simulink model "analysis_PI_ctrl_lin_model_z"  (R2020b)
settings: Solver=VariableStepAuto  StartTime=0.0  StopTime=10.0  RelTol=1e-3
values from neighbouring files (symbols this model uses):
  B = 10    [hinfCostFunc.m]    (also in hinf_analysis_z.m; hinf_cmd_lmi.m = [zeros(4,2); Sigma.B]; init_rob_synth_sim.m; muCostFunc.m = 11)
  dq0 = [0;0;0]    [hinfCostFunc.m]    (also in hinf_analysis_z.m; init_rob_synth_sim.m = [0; 0; 0]; muCostFunc.m; mu_analysis_z.m)
  ev0 = [0;0;0]    [hinfCostFunc.m]    (also in hinf_analysis_z.m; muCostFunc.m; mu_analysis_z.m)
  K = 150    [hinfCostFunc.m]    (also in hinf_analysis_z.m; init_rob_synth_sim.m; muCostFunc.m = ureal('K',160,'Percentage',50); mu_analysis_z.m = ureal('K',160,'Percentage',50))
  Ki = 0.08    [hinfCostFunc.m]    (also in hinf_analysis_z.m; muCostFunc.m; mu_analysis_z.m; robust_synthesis.m)
  Kp = 0.015    [hinfCostFunc.m]    (also in hinf_analysis_z.m; muCostFunc.m; mu_analysis_z.m; robust_synthesis.m)
  M = 0.45    [hinfCostFunc.m]    (also in hinf_analysis_z.m; init_rob_synth_sim.m; muCostFunc.m = 0.42; mu_analysis_z.m = 0.42)
  q0 = [1.676; -4.363; 1.497]    [hinfCostFunc.m]    (also in hinf_analysis_z.m; init_rob_synth_sim.m; muCostFunc.m; mu_analysis_z.m)
  Sigma = minreal(Sigma, [], false)    [hinfCostFunc.m]    (also in hinf_analysis_z.m = youbot_lin_model_ss_z; hinf_cmd_lmi.m = youbot_lin_model_ss_z; muCostFunc.m; mu_analysis_z.m = youbot_lin_model_ss_z)
  tau_m = 1/(10*2*pi)    (= 0.0159154943092)    [hinfCostFunc.m]    (also in hinf_analysis_z.m; init_rob_synth_sim.m; muCostFunc.m; mu_analysis_z.m)
settings Model: Creator=fortineau_vin  LastModifiedBy=fortineau_vin

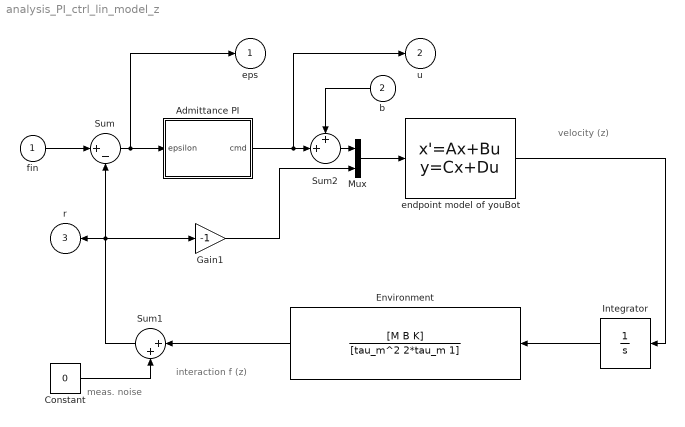
== system analysis_PI_ctrl_lin_model_z ==
  note: velocity (z)
  note: interaction f (z)
  note: meas. noise
  fin : Inport  PortDimensions=1
  b : Inport  Port=2  PortDimensions=1
  Admittance PI : Subsystem
  Constant : Constant  Value=0
  Environment : TransferFcn  Numerator=[M B K]  Denominator=[tau_m^2 2*tau_m 1]
  Gain1 : Gain  Gain=-1
  Integrator : Integrator
  Mux : Mux  Inputs=2
  Sum : Sum  Inputs=|+-
  Sum1 : Sum  Inputs=|++
  Sum2 : Sum  Inputs=++|
  endpoint model of youBot : StateSpace  A=Sigma.A  B=Sigma.B  C=Sigma.C  D=Sigma.D  InitialCondition=[q0;dq0;ev0]
  eps : Outport  PortDimensions=1
  u : Outport  Port=2  PortDimensions=1
  r : Outport  Port=3  PortDimensions=1
  wires:
  Sum/1 -> eps/1, Admittance PI/1(epsilon)
  Mux/1 -> endpoint model of youBot/1
  fin/1 -> Sum/1
  Admittance PI/1(cmd) -> Sum2/2, u/1
  Integrator/1 -> Environment/1
  endpoint model of youBot/1 -> Integrator/1
  Environment/1 -> Sum1/1
  Sum1/1 -> Sum/2, Gain1/1, r/1
  Constant/1 -> Sum1/2
  Sum2/1 -> Mux/1
  b/1 -> Sum2/1
  Gain1/1 -> Mux/2

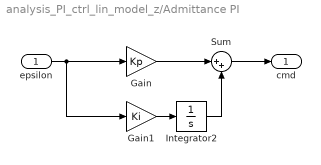
== system analysis_PI_ctrl_lin_model_z/Admittance PI ==
  epsilon : Inport
  Gain : Gain  Gain=Kp
  Gain1 : Gain  Gain=Ki
  Integrator2 : Integrator
  Sum : Sum  Inputs=|++
  cmd : Outport  VectorParamsAs1DForOutWhenUnconnected=off
  wires:
  Integrator2/1 -> Sum/2
  Gain/1 -> Sum/1
  Gain1/1 -> Integrator2/1
  epsilon/1 -> Gain/1, Gain1/1
  Sum/1 -> cmd/1
